simulink model "lin_mod"  (Simulink 6.4)
settings: Solver=ode45  StartTime=0.0  StopTime=10.0  RelTol=1e-3
settings Model: LastModifiedBy=kookmin

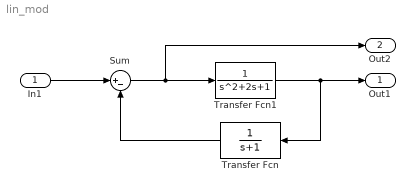
== system lin_mod ==
  In1 : Inport
  Sum : Sum  Inputs=|+-
  Transfer Fcn : TransferFcn  Orientation=left  Denominator=[1 1]
  Transfer Fcn1 : TransferFcn
  Out1 : Outport
  Out2 : Outport  Port=2
  wires:
  In1/1 -> Sum/1
  Sum/1 -> Transfer Fcn1/1, Out2/1
  Transfer Fcn1/1 -> Out1/1, Transfer Fcn/1
  Transfer Fcn/1 -> Sum/2
